simulink model "papershowcase"  (R2014a)
settings: Solver=FixedStepDiscrete  StartTime=0.0  StopTime=10.0  FixedStep=1  RelTol=1e-3
settings Model: Creator=Administrator  LastModifiedBy=Administrator

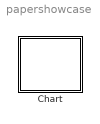
== system papershowcase ==
  Chart : Stateflow chart  TreatAsAtomicUnit=on

== stateflow chart papershowcase/Chart ==
  state Container
    entry:x= int32(0);y= int32(1);CLK= int32(0);z= int32(0);result=false;
    during:CLK=CLK+1;
    state B [parallel]
      settings: executionOrder=2
      state B3
      state BCount
        entry:result=true;
        state B2
        (default) -> B2
      state B1
      (junction 49) -> B3 [order 1] : [y>=10]
      B1 -> (junction 49) : switch_on{x=x+1;}/{y=y-3;}
      (junction 49) -> B2 [order 2] : [x==3]/{z= x/y}
      (default) -> B1
    state C [parallel]
      settings: executionOrder=3
      state C1
      state C2
      (default) -> C1
      C1 -> C2 : [result]
    state A [parallel]
      settings: executionOrder=1
      state A1
      state A2
      (default) -> A1
      A1 -> A2 : [after(2,sec)]/{switch_on}
      A2 -> A1 : {y=y+1}
  (default) -> Container
  data: x local int32 =0; CLK local int32 =0; result local boolean =false; y local int32 =1; z local int32 =0
  events: switch_on local FUNCTION_CALL_EVENT; switch_off local FUNCTION_CALL_EVENT
